simulink model "MotionController"  (R2021a)
settings: Solver=VariableStepAuto  StartTime=0.0  StopTime=10.0  RelTol=1e-3
settings Model: DataDictionary=robotDD.sldd  Creator=Highlander  LastModifiedBy=Highlander

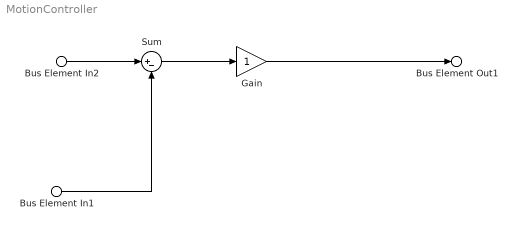
== system MotionController ==
  Bus Element In1 : Inport  PortName=SensorData
  Bus Element In2 : Inport  Port=2  PortName=TargetPosition
  Gain : Gain
  Sum : Sum  Inputs=|+-
  Bus Element Out1 : Outport  PortName=Command
  wires:
  Bus Element In2/1 -> Sum/1
  Bus Element In1/1 -> Sum/2
  Sum/1 -> Gain/1
  Gain/1 -> Bus Element Out1/1
